simulink library "SLUGS_Library"  (Simulink 7.8)
settings: Solver=ode45  SolverMode=SingleTasking  StartTime=0.0  StopTime=10.0  RelTol=1e-3
values from neighbouring files (symbols this model uses):
  apSampleTime = 0.01    [mcuInit.m]
  derivativesConstant = 5    [mcuInit.m]
  latlong_WP = 1    [mcuInit.m]
  T = 0.01    [mcuInit.m]
  Xpoints = [0 0]    [mcuInit.m]
  Ypoints = [0 0]    [mcuInit.m]
  Zpoints = [0 0]    [mcuInit.m]
undefined symbols (not defined in the file or in its folder): bankCommandLimit, barAdjust, baroCutTemp, baroOffset, baroScale, barTGain1, barTGain2, barTMean1, barTMean2, baseHeight, baseTemp, daLimit, deLimit, DiscIntNeverNeededParam, drLimit, dtLimit, gaind, getGSLocation, getWP, GS_location, Init_onlyOnce, Init_Reset, IPStar, ISA_g, lapseRate, mass, maxAcc, MaxDwnPthStar, maxDynPressure, maxEta, Ndelay, param, pitAdjust, pitchCommandLimit, pitCutTemp, pitotOffset, pitotScale, pitTGain1, pitTGain2, pitTMean1, pitTMean2, polesd, pressureSensorCutoff, rollControlLimit, SampleT, setDiagnosticFloat, setDiagnosticShort, setLogFloat1, setLogFloat2, setNavLong, setNavNav, tanIntercept, Ts, u1, y1, yawDamperLimit, yo, zerosd
libraries: SLUGS_Library x90, simulink x37, dsPICdrivers x33, aerolibconvert2 x4, aerolibutil x1, aerolibobsolete x1
(part 4 of 7)

== system SLUGS_Library/InnerLoop/Longitudinal Channel/Protect NaNs2 ==
  In1 : Inport
  Integer Delay3 : Delay  DelayLength=1  InputProcessing=Inherited  SampleTime=T
  Relational Operator2 : RelationalOperator  Operator===  OutDataTypeStr=uint(8)
  Switch3 : Switch  Criteria=u2 > Threshold  Threshold=0.3  SampleTime=.01
  Out1 : Outport
  wires:
  Relational Operator2/1 -> Switch3/2
  In1/1 -> Switch3/1, Relational Operator2/1, Relational Operator2/2
  Switch3/1 -> Integer Delay3/1, Out1/1
  Integer Delay3/1 -> Switch3/3

== system SLUGS_Library/InnerLoop/Longitudinal Channel/Protect NaNs3 ==
  In1 : Inport
  Integer Delay3 : Delay  DelayLength=1  InputProcessing=Inherited  SampleTime=T
  Relational Operator2 : RelationalOperator  Operator===  OutDataTypeStr=uint(8)
  Switch3 : Switch  Criteria=u2 > Threshold  Threshold=0.3  SampleTime=.01
  Out1 : Outport
  wires:
  Relational Operator2/1 -> Switch3/2
  In1/1 -> Switch3/1, Relational Operator2/1, Relational Operator2/2
  Switch3/1 -> Integer Delay3/1, Out1/1
  Integer Delay3/1 -> Switch3/3

== system SLUGS_Library/InnerLoop/Longitudinal Channel/Protect NaNs4 ==
  In1 : Inport
  Integer Delay3 : Delay  DelayLength=1  InputProcessing=Inherited  SampleTime=T
  Relational Operator2 : RelationalOperator  Operator===  OutDataTypeStr=uint(8)
  Switch3 : Switch  Criteria=u2 > Threshold  Threshold=0.3  SampleTime=.01
  Out1 : Outport
  wires:
  Relational Operator2/1 -> Switch3/2
  In1/1 -> Switch3/1, Relational Operator2/1, Relational Operator2/2
  Switch3/1 -> Integer Delay3/1, Out1/1
  Integer Delay3/1 -> Switch3/3

== system SLUGS_Library/InnerLoop/Longitudinal Channel/Subsystem5 ==
  u : Inport
  C Function Call1 : dsPICdrivers/OTHERS/C Function Call  Tag=dsPIC_dsPIC_CFunctionCall  FctUpdate=Output Function  fctName='myCos'  INPUT_SIZE=1  INPUT1=real32  INPUT2=--  INPUT3=--  OUTPUT_SIZE=1  OUTPUT1=real32  SampleTime=-1  InputType=[ 7 ]  OutputType=[ 7 ]  FctDeclaration=extern real32_T myCos(real32_T u1);  FctCall=%y1 = myCos(%u1);  OrderingInOutPopup=None  FctStart=None  FctStart_Name=Init_onlyOnce  FctStart_Declaration=inline extern void Init_onlyOnce();  FctStart_Call=Init_onlyOnce();  FctInit=None  FctInit_Name=Init_Reset  FctInit_Declaration=inline extern void Init_Reset();  FctInit_Call=Init_Reset();  PinDigitalInput=[]  PinDigitalOutput=[]  AnalogueInput=[]
  cos(u) : Outport
  wires:
  C Function Call1/1 -> cos(u)/1
  u/1 -> C Function Call1/1

== system SLUGS_Library/InnerLoop/Navigation/Compute WP Index ==
  T1 : Inport
  Puav : Inport  Port=2
  Max WP Index : Inport  Port=3
  StartingWP : Inport  Port=4
  "WP1 " : Inport  Port=5
  R : Inport  Port=6
  WP Fly : Inport  Port=7
  Add : Sum  Inputs=2
  Compute Distance : SLUGS_Library/Navigation/Compute Distance
  Compute Modified L1 : Subsystem
  Data Type Conversion : DataTypeConversion  OutDataTypeStr=double  SampleTime=apSampleTime
  Data Type Conversion1 : DataTypeConversion  OutDataTypeStr=double  SampleTime=apSampleTime
  Embedded MATLAB Function : MATLAB Function  TreatAsAtomicUnit=on
  Enabled Subsystem : Subsystem  TreatAsAtomicUnit=on
  Hit  Crossing : HitCross  HitCrossingOffset=0.9  HitCrossingDirection=rising  SampleTime=apSampleTime
  IC : InitialCondition
  IC1 : InitialCondition  Value=0
  Integer Delay : Delay  DelayLength=1  InputProcessing=Inherited
  Integer Delay2 : Delay  DelayLength=1  InitialCondition=0  InputProcessing=Inherited
  Integer Delay3 : Delay  DelayLength=1  InitialCondition=150  InputProcessing=Inherited
  Logical Operator : Logic  Operator=OR  AllPortsSameDT=off  OutDataTypeStr=boolean
  "Puav " : InportShadow  Port=2
  Subsystem : Subsystem
  Switch Distance Less than? : RelationalOperator  OutDataTypeStr=boolean  SampleTime=apSampleTime
  WP1 1 : InportShadow  Port=5
  WP Change : Outport
  WP0 : Outport  Port=2
  WP1 : Outport  Port=3
  UAV IC : Outport  Port=4
  wires:
  [WpEnabl] -> Logical Operator/2
  Logical Operator/1 -> WP Change/1
  [WpEnabl] -> Embedded MATLAB Function/4(wpEnabl)
  IC1/1 -> Subsystem/1(WP Fly)
  Enabled Subsystem/1(Out1) -> UAV IC/1
  "Puav "/1 -> Enabled Subsystem/1(In1)
  Subsystem/1(Just Enab) -> [WpEnabl], Enabled Subsystem/Enable
  WP Fly/1 -> Data Type Conversion1/1
  R/1 -> Compute Modified L1/4(R)
  Integer Delay3/1 -> Switch Distance Less than?/1
  Compute Modified L1/1(P) -> Integer Delay3/1
  IC/1 -> Integer Delay2/1, Add/2
  Add/1 -> Logical Operator/1, Compute Modified L1/Enable
  Integer Delay2/1 -> Add/1
  T1/1 -> Compute Modified L1/2(T1)
  WP1 1/1 -> Compute Modified L1/1(WP1)
  Embedded MATLAB Function/3(wp2) -> Compute Modified L1/3(WP2)
  Data Type Conversion/1 -> Hit  Crossing/1
  Hit  Crossing/1 -> IC/1, Embedded MATLAB Function/3(swIncrement)
  "WP1 "/1 -> Integer Delay/1
  Compute Distance/1 -> Switch Distance Less than?/2
  Max WP Index/1 -> Embedded MATLAB Function/2(wpCount)
  Switch Distance Less than?/1 -> Data Type Conversion/1
  StartingWP/1 -> Embedded MATLAB Function/1(wpStart)
  Embedded MATLAB Function/1(wp0) -> WP0/1
  Embedded MATLAB Function/2(wp1) -> WP1/1
  Puav/1 -> Compute Distance/1
  Integer Delay/1 -> Compute Distance/2  "next WP"
  Data Type Conversion1/1 -> IC1/1

== system SLUGS_Library/InnerLoop/Navigation/Get Wps Compute Frenet ==
  WP Idx 0 : Inport
  WP Idx 1 : Inport  Port=2
  UAV IC : Inport  Port=3
  Enable : EnablePort
  Compute Frenet : SLUGS_Library/Navigation/Compute Frenet
  Switch : Switch  Criteria=u2 > Threshold  Threshold=0.3
  get WP Coord from Index : SLUGS_Library/Navigation/get WP Coord from Index
  "get WP Coord from Index " : SLUGS_Library/Navigation/get WP Coord from Index
  T : Outport
  N : Outport  Port=2
  WP 1 : Outport  Port=3
  wires:
  WP Idx 0/1 -> get WP Coord from Index/1, Switch/2
  Compute Frenet/1 -> T/1
  Compute Frenet/2 -> N/1
  WP Idx 1/1 -> "get WP Coord from Index "/1
  "get WP Coord from Index "/1 -> Compute Frenet/2, WP 1/1
  Switch/1 -> Compute Frenet/1
  get WP Coord from Index/1 -> Switch/1
  UAV IC/1 -> Switch/3

== system SLUGS_Library/Navigation/Compute WP Index/Compute Modified L1 ==
  WP1 : Inport
  T1 : Inport  Port=2
  WP2 : Inport  Port=3
  R : Inport  Port=4
  Enable : EnablePort  ShowOutputPort=on
  Compute T  in Frenet : Subsystem  AncestorBlock=SLUGS_Library/Navigation/Compute Frenet
  Get Circles : Subsystem
  Integer Delay1 : Delay  DelayLength=1  InputProcessing=Inherited
  Integer Delay2 : Delay  DelayLength=1  InputProcessing=Inherited
  To Workspace : ToWorkspace  VariableName=wpChange  SampleTime=-1  SaveFormat=Structure
  WP1_1 : InportShadow  Port=1
  get WP Coord from Index : SLUGS_Library/Navigation/get WP Coord from Index
  P : Outport
  wires:
  get WP Coord from Index/1 -> Integer Delay2/1
  Integer Delay2/1 -> Compute T  in Frenet/2(Pos 2)
  Compute T  in Frenet/1(T) -> Get Circles/2(T2)
  WP1/1 -> Compute T  in Frenet/1(Pos 1)
  WP2/1 -> get WP Coord from Index/1
  T1/1 -> Integer Delay1/1
  Get Circles/1(P) -> P/1
  WP1_1/1 -> Get Circles/3("Wp_to ")
  Integer Delay1/1 -> Get Circles/1(T1)
  Enable/1 -> To Workspace/1
  R/1 -> Get Circles/4(R)

== system SLUGS_Library/Navigation/Compute WP Index/Enabled Subsystem ==
  In1 : Inport
  Enable : EnablePort
  Out1 : Outport
  wires:
  In1/1 -> Out1/1

== system SLUGS_Library/Navigation/Compute WP Index/Subsystem ==
  WP Fly : Inport
  Add1 : Sum  Inputs=2
  Hit  Crossing1 : HitCross  HitCrossingOffset=0.3  HitCrossingDirection=rising  SampleTime=apSampleTime
  Integer Delay1 : Delay  DelayLength=1  InitialCondition=0  InputProcessing=Inherited
  Just Enab : Outport
  wires:
  Integer Delay1/1 -> Add1/1
  Hit  Crossing1/1 -> Add1/2, Integer Delay1/1
  Add1/1 -> Just Enab/1
  WP Fly/1 -> Hit  Crossing1/1

== system SLUGS_Library/Navigation/Geod2LTP/ECEF2LTP (UEN) ==
  ECEF coordinates : Inport
  "Long, Lat" : Inport  Port=2
  Deg2R : Gain  Gain=pi/180  SaturateOnIntegerOverflow=on  OutDataTypeStr=Inherit: Same as input  ParamDataTypeStr=Inherit: Same as input
  Demux3 : Demux  Outputs=2
  From Body to Universal1 : Subsystem
  Product1 : Product  Multiplication=Matrix(*)  SaturateOnIntegerOverflow=on  InputSameDT=on  OutDataTypeStr=Inherit: Same as first input
  Out : Outport
  wires:
  From Body to Universal1/1(DCM) -> Product1/1
  ECEF coordinates/1 -> Product1/2
  Deg2R/1 -> Demux3/1
  Demux3/1 -> From Body to Universal1/1(long)
  Demux3/2 -> From Body to Universal1/2(lat)
  Product1/1 -> Out/1
  "Long, Lat"/1 -> Deg2R/1

== system SLUGS_Library/Navigation/Geod2LTP/Geod2ECEF1 ==
  "height, m" : Inport
  "lat, deg" : Inport  Port=2
  lon,deg : Inport  Port=3
  (Rh+h)cos(phi)*cos(lamb)=Xe : Product  Inputs=3  OutDataTypeStr=single  SaturateOnIntegerOverflow=on  InputSameDT=on
  (Rh+h)cos(phi)*sin(lamb)=Ye : Product  Inputs=3  OutDataTypeStr=single  SaturateOnIntegerOverflow=on  InputSameDT=on
  Deg2R : Gain  Gain=pi/180  OutDataTypeStr=float('single')  SaturateOnIntegerOverflow=on  ParamDataTypeStr=Inherit: Same as input
  Deg2R1 : Gain  Gain=pi/180  OutDataTypeStr=float('single')  SaturateOnIntegerOverflow=on  ParamDataTypeStr=Inherit: Same as input
  Product1 : Product  SaturateOnIntegerOverflow=on  InputSameDT=on  OutDataTypeStr=Inherit: Same as first input
  Re=equatorial radius : Constant  Value=Re  OutDataTypeStr=single
  Rh : Product  Inputs=*/  OutDataTypeStr=single  SaturateOnIntegerOverflow=on  InputSameDT=on
  Rh(1-e^2) : Product  OutDataTypeStr=single  SaturateOnIntegerOverflow=on  InputSameDT=on
  Sum1 : Sum  Inputs=+-|  SaturateOnIntegerOverflow=on  InputSameDT=on  OutDataTypeStr=Inherit: Same as first input
  Sum2 : Sum  SaturateOnIntegerOverflow=on  InputSameDT=on  OutDataTypeStr=Inherit: Same as first input
      settings: AttributesFormatString=Rh+h
  Sum3 : Sum  Inputs=|+-  SaturateOnIntegerOverflow=on  InputSameDT=on  OutDataTypeStr=Inherit: Same as first input
  Sum4 : Sum  OutDataTypeStr=single  SaturateOnIntegerOverflow=on  InputSameDT=on
      settings: AttributesFormatString=(1-e^2)Rh+h
  Ze : Product  OutDataTypeStr=single  SaturateOnIntegerOverflow=on  InputSameDT=on
  const : Constant  OutDataTypeStr=single
  const1 : Constant  OutDataTypeStr=single
  cos(lamb) : Trigonometry  Operator=cos
  cos(phi) : Trigonometry  Operator=cos
  eccentricity^2 : Subsystem
  f : Fcn  Expr=sqrt(u(1))
  sin(lamb) : Trigonometry
  sin(phi) : Trigonometry
  sin(phi)^2 : Product  SaturateOnIntegerOverflow=on  InputSameDT=on  OutDataTypeStr=Inherit: Same as first input
  "Xe, m " : Outport
  "Ye, m " : Outport  Port=2
  "Ze, m " : Outport  Port=3
  wires:
  (Rh+h)cos(phi)*sin(lamb)=Ye/1 -> "Ye, m "/1
  (Rh+h)cos(phi)*cos(lamb)=Xe/1 -> "Xe, m "/1
  Sum2/1 -> (Rh+h)cos(phi)*cos(lamb)=Xe/1, (Rh+h)cos(phi)*sin(lamb)=Ye/1
  Deg2R1/1 -> sin(lamb)/1, cos(lamb)/1
  Deg2R/1 -> sin(phi)/1, cos(phi)/1
  Ze/1 -> "Ze, m "/1
  sin(lamb)/1 -> (Rh+h)cos(phi)*sin(lamb)=Ye/3
  cos(lamb)/1 -> (Rh+h)cos(phi)*cos(lamb)=Xe/3
  cos(phi)/1 -> (Rh+h)cos(phi)*sin(lamb)=Ye/2, (Rh+h)cos(phi)*cos(lamb)=Xe/2
  lon,deg/1 -> Deg2R1/1
  Sum4/1 -> Ze/2
  Rh(1-e^2)/1 -> Sum4/1
  Sum3/1 -> Rh(1-e^2)/1  "1-e^2"
  const1/1 -> Sum3/1
  sin(phi)^2/1 -> Product1/2
  eccentricity^2/1(e^2) -> Sum3/2, Product1/1
  "height, m"/1 -> Sum2/1, Sum4/2
  const/1 -> Sum1/1
  Sum1/1 -> f/1
  Product1/1 -> Sum1/2
  Rh/1 -> Rh(1-e^2)/2, Sum2/2
  Re=equatorial radius/1 -> Rh/1
  f/1 -> Rh/2
  sin(phi)/1 -> Ze/1, sin(phi)^2/2, sin(phi)^2/1
  "lat, deg"/1 -> Deg2R/1

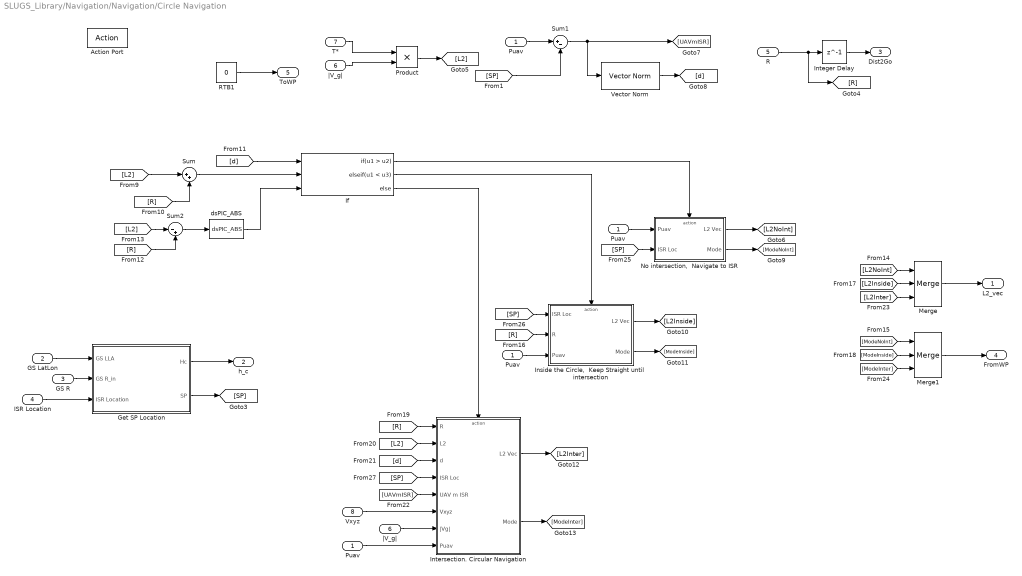
== system SLUGS_Library/Navigation/Navigation/Circle Navigation ==
  Puav : Inport
  GS LatLon : Inport  Port=2
  GS R : Inport  Port=3
  ISR Location : Inport  Port=4
  R : Inport  Port=5
  |V_g| : Inport  Port=6
  T* : Inport  Port=7
  Vxyz : Inport  Port=8
  Action Port : ActionPort
  Get SP Location : Subsystem
  If : If  NumInputs=3  IfExpression=u1 > u2  ElseIfExpressions=u1 < u3
  "Inside the Circle,  Keep Straight until  intersection" : Subsystem  TreatAsAtomicUnit=on
  Integer Delay : Delay  DelayLength=1  InputProcessing=Inherited
  Intersection. Circular Navigation : Subsystem  TreatAsAtomicUnit=on
  Merge : Merge  Inputs=3
  Merge1 : Merge  Inputs=3
  "No intersection,  Navigate to ISR" : Subsystem  TreatAsAtomicUnit=on
  Product : Product  OutDataTypeStr=single  RndMeth=Zero
  "Puav   " : InportShadow  Port=1
  "Puav    " : InportShadow  Port=1
  "Puav     " : InportShadow  Port=1
  RTB1 : Constant  Value=0  OutDataTypeStr=uint8
  Sum : Sum  Inputs=|++
  Sum1 : Sum  Inputs=|+-
  Sum2 : Sum  Inputs=|-+
  Vector Norm : SLUGS_Library/Vector Norm
  dsPIC_ABS : SLUGS_Library/dsPIC_ABS
  "|V_g| " : InportShadow  Port=6
  L2_vec : Outport
  h_c : Outport  Port=2
  Dist2Go : Outport  Port=3
  FromWP : Outport  Port=4  InitialOutput=[1]
  ToWP : Outport  Port=5  InitialOutput=[1]
  wires:
  "Puav     "/1 -> Intersection. Circular Navigation/8(Puav)
  Get SP Location/1(Hc) -> h_c/1
  [ModeInter] -> Merge1/3
  [L2Inter] -> Merge/3
  "|V_g| "/1 -> Intersection. Circular Navigation/7(|Vg|)
  Vxyz/1 -> Intersection. Circular Navigation/6(Vxyz)
  [UAVmISR] -> Intersection. Circular Navigation/5(UAV m ISR)
  [SP] -> Intersection. Circular Navigation/4(ISR Loc)
  [d] -> Intersection. Circular Navigation/3(d)
  [L2] -> Intersection. Circular Navigation/2(L2)
  [R] -> Intersection. Circular Navigation/1(R)
  Intersection. Circular Navigation/2(Mode) -> [ModeInter]
  Intersection. Circular Navigation/1(L2 Vec) -> [L2Inter]
  Puav/1 -> "Inside the Circle,  Keep Straight until  intersection"/3(Puav)
  [ModeInside] -> Merge1/2
  [L2Inside] -> Merge/2
  "Inside the Circle,  Keep Straight until  intersection"/2(Mode) -> [ModeInside]
  "Inside the Circle,  Keep Straight until  intersection"/1(L2 Vec) -> [L2Inside]
  [R] -> "Inside the Circle,  Keep Straight until  intersection"/2(R)
  [SP] -> "Inside the Circle,  Keep Straight until  intersection"/1(ISR Loc)
  [ModeNoInt] -> Merge1/1
  [L2NoInt] -> Merge/1
  "No intersection,  Navigate to ISR"/2(Mode) -> [ModeNoInt]
  "No intersection,  Navigate to ISR"/1(L2 Vec) -> [L2NoInt]
  [SP] -> "No intersection,  Navigate to ISR"/2(ISR Loc)
  "Puav    "/1 -> "No intersection,  Navigate to ISR"/1(Puav)
  If/3 -> Intersection. Circular Navigation/Action
  If/2 -> "Inside the Circle,  Keep Straight until  intersection"/Action
  If/1 -> "No intersection,  Navigate to ISR"/Action
  Merge/1 -> L2_vec/1
  dsPIC_ABS/1 -> If/3
  Sum2/1 -> dsPIC_ABS/1
  [R] -> Sum2/2
  [L2] -> Sum2/1
  Sum/1 -> If/2
  [d] -> If/1
  Vector Norm/1 -> [d]
  Sum1/1 -> [UAVmISR], Vector Norm/1
  [SP] -> Sum1/2
  "Puav   "/1 -> Sum1/1
  [R] -> Sum/2
  [L2] -> Sum/1
  RTB1/1 -> ToWP/1
  T*/1 -> Product/1
  |V_g|/1 -> Product/2
  Product/1 -> [L2]
  Get SP Location/2(SP) -> [SP]
  GS LatLon/1 -> Get SP Location/1(GS LLA)
  GS R/1 -> Get SP Location/2(GS R_in)
  ISR Location/1 -> Get SP Location/3(ISR Location)
  Integer Delay/1 -> Dist2Go/1
  R/1 -> Integer Delay/1, [R]
  Merge1/1 -> FromWP/1

== system SLUGS_Library/Navigation/Navigation/Get 2D Groundspeed ==
  Vxyz : Inport  SampleTime=apSampleTime
  Vector Norm : SLUGS_Library/Vector Norm
  |V_g| : Outport
  wires:
  Vector Norm/1 -> |V_g|/1
  Vxyz/1 -> Vector Norm/1

== system SLUGS_Library/Navigation/Navigation/L2+ ==
  |V_g| : Inport
  L2_vec : Inport  Port=2
  Vxyz : Inport  Port=3
  T*(m) : Inport  Port=4
  Constant10 : Constant  Value=maxEta  OutDataTypeStr=single
  "Get Sin, Cos eta" : Subsystem
  L2+ : Subsystem
  Rad2Deg : Gain  Gain=180/pi
  Relational Operator : RelationalOperator  Operator=<=  OutDataTypeStr=boolean
  Subsystem : Subsystem
  Switch : Switch  Criteria=u2 > Threshold  Threshold=0.3
  dsPIC_ABS : SLUGS_Library/dsPIC_ABS
  dsPIC_atan2 : SLUGS_Library/dsPIC_atan2
  "if sin(eta) < 0 - maxAcc else                 maxAcc " : Subsystem
  "|V_g| " : InportShadow  Port=1
  phi_c : Outport
  eta : Outport  Port=2
  wires:
  Rad2Deg/1 -> eta/1
  Subsystem/1(phi_c) -> phi_c/1
  T*(m)/1 -> L2+/3(T*)
  "|V_g| "/1 -> L2+/2(|V_g|)
  "Get Sin, Cos eta"/1(sin(eta)) -> L2+/1(sin(eta)), dsPIC_atan2/1, "if sin(eta) < 0 - maxAcc else                 maxAcc "/1(sin(eta))
  "Get Sin, Cos eta"/2(cos(eta)) -> dsPIC_atan2/2
  dsPIC_atan2/1 -> Rad2Deg/1, dsPIC_ABS/1  "eta"
  dsPIC_ABS/1 -> Relational Operator/1
  Constant10/1 -> Relational Operator/2
  Relational Operator/1 -> Switch/2
  L2+/1(a_c) -> Switch/1
  "if sin(eta) < 0 - maxAcc else                 maxAcc "/1(+ - maxAcc) -> Switch/3
  Switch/1 -> Subsystem/1(a_c)
  |V_g|/1 -> "Get Sin, Cos eta"/1(|V_g|)
  L2_vec/1 -> "Get Sin, Cos eta"/2(L2_vec)
  Vxyz/1 -> "Get Sin, Cos eta"/3(Vxyz)

== system SLUGS_Library/Navigation/Navigation/Line Segment ==
  Puav : Inport
  MidLvl h_c : Inport  Port=2
  Action Port : ActionPort
  Gain : Gain  Gain=-1
  Gain1 : Gain  Gain=-1
  "Puav " : InportShadow  Port=1
  RTB : Constant  Value=0  OutDataTypeStr=uint8
  RTB1 : Constant  Value=0  OutDataTypeStr=uint8
  Vector Norm : SLUGS_Library/Vector Norm
  L2_vec : Outport
  h_c : Outport  Port=2
  Dist2Go : Outport  Port=3
  FromWP : Outport  Port=4  InitialOutput=[1]
  ToWP : Outport  Port=5  InitialOutput=[2]
  wires:
  Gain/1 -> L2_vec/1
  Puav/1 -> Gain/1
  MidLvl h_c/1 -> h_c/1
  Vector Norm/1 -> Dist2Go/1
  RTB/1 -> FromWP/1
  "Puav "/1 -> Gain1/1
  Gain1/1 -> Vector Norm/1
  RTB1/1 -> ToWP/1

== system SLUGS_Library/Navigation/Navigation/Minimum Turn Radius ==
  U_c : Inport
  Scale Factor : Inport  Port=2
  Constant1 : Constant  Value=maxAcc  OutDataTypeStr=single
  IC : InitialCondition  Value=1.5
  Product1 : Product  RndMeth=Zero
  Product2 : Product  RndMeth=Zero
  Product3 : Product  Inputs=*/  RndMeth=Zero
  "[1.5 10]" : Saturate  UpperLimit=10  LowerLimit=1.5
  R : Outport
  wires:
  U_c/1 -> Product1/2, Product1/1
  Product2/1 -> Product3/1
  Constant1/1 -> Product3/2
  Product1/1 -> Product2/2
  Scale Factor/1 -> IC/1
  Product3/1 -> R/1
  "[1.5 10]"/1 -> Product2/1
  IC/1 -> "[1.5 10]"/1

== system SLUGS_Library/Navigation/Navigation/Normal WP  Navigation ==
  wpEnable : Inport
  GS_LatLon : Inport  Port=2
  GS_R_in : Inport  Port=3
  |V_g| : Inport  Port=4
  T* : Inport  Port=5
  Puav : Inport  Port=6
  TurnLeadTime : Inport  Port=7
  MaxWp : Inport  Port=8
  Action Port : ActionPort
  Add : Sum  Inputs=+-
  Compute WP Switching Trigger : Subsystem
  Constant1 : Constant  OutDataTypeStr=boolean  SampleTime=0.01
  Constant2 : Constant  OutDataTypeStr=boolean  SampleTime=0.01
  Embedded MATLAB Function : MATLAB Function  TreatAsAtomicUnit=on
  "GS_LatLon " : InportShadow  Port=2
  "GS_R_in " : InportShadow  Port=3
  Gain : Gain  Gain=0.4
  Get Frenet : Subsystem
  IC : InitialCondition  Value=0
  Integer Delay : Delay  DelayLength=1  InitialCondition=1  InputProcessing=Inherited
  On WP Enable : Subsystem  TreatAsAtomicUnit=on
  Product : Product  OutDataTypeStr=single  RndMeth=Zero
  "Puav " : InportShadow  Port=6
  Relational Operator : RelationalOperator  Operator=>  OutDataTypeStr=boolean
  Switch : Switch  Criteria=u2 > Threshold  Threshold=0.3  ZeroCross=off
  Switch1 : Switch  Criteria=u2 > Threshold  Threshold=0.3  ZeroCross=off
  To Workspace : ToWorkspace  VariableName=IP  SampleTime=-1  SaveFormat=Array
  To Workspace1 : ToWorkspace  VariableName=L2Vec  SampleTime=-1  SaveFormat=Array
  To Workspace2 : ToWorkspace  VariableName=AimPointVect  SampleTime=-1  SaveFormat=Array
  To Workspace3 : ToWorkspace  VariableName=IPReached  SampleTime=-1  SaveFormat=Array
  Vector Norm : SLUGS_Library/Vector Norm
  Zero out Z2 : MATLAB Function  TreatAsAtomicUnit=on
  computeCurrentWP : MATLAB Function  TreatAsAtomicUnit=on
  "|V_g| " : InportShadow  Port=4
  L2_vec : Outport
  h_c : Outport  Port=2
  Dist2Go : Outport  Port=3
  FromWP : Outport  Port=4  InitialOutput=[1]
  ToWP : Outport  Port=5  InitialOutput=[2]
  wires:
  IC/1 -> Switch/2, To Workspace3/1, [IPReached]
  [L2] -> Compute WP Switching Trigger/6(L2)
  MaxWp/1 -> computeCurrentWP/2(maxWp)
  computeCurrentWP/2(WP1) -> Get Frenet/4(To WP), ToWP/1
  computeCurrentWP/1(WP0) -> Get Frenet/3(From WP), FromWP/1
  Compute WP Switching Trigger/1(Switch) -> Integer Delay/1
  Compute WP Switching Trigger/3(L2Vec) -> To Workspace1/1, Switch/1
  Get Frenet/4(N1) -> Compute WP Switching Trigger/3(N1)
  Get Frenet/5(TurnLeadDistance) -> Compute WP Switching Trigger/4(LeadDistance)
  TurnLeadTime/1 -> Get Frenet/5(TurnLeadTime)
  "|V_g| "/1 -> Get Frenet/6(|V_g|)
  "Puav "/1 -> Add/2
  Puav/1 -> Compute WP Switching Trigger/5(Puav)
  Get Frenet/3(T1) -> Compute WP Switching Trigger/2(T1)
  Get Frenet/2(ToWp) -> Compute WP Switching Trigger/1(ToWp)
  "GS_R_in "/1 -> Get Frenet/2(GS R_in)
  "GS_LatLon "/1 -> Get Frenet/1(GS LLA)
  Embedded MATLAB Function/1(reached) -> IC/1
  Switch/1 -> L2_vec/1
  Relational Operator/1 -> Embedded MATLAB Function/2(didReachIP)
  Vector Norm/1 -> Relational Operator/2, [dist2AP]  "Dist2AimPoint"
  Gain/1 -> Relational Operator/1
  [L2] -> Gain/1
  Add/1 -> To Workspace2/1, Switch/3, Vector Norm/1  "Pa = HP - Pned"
  Zero out Z2/1(P) -> Add/1
  On WP Enable/1(P_i) -> To Workspace/1, Zero out Z2/1(Pin)  "WP0 - L2*IP*T1"
  GS_R_in/1 -> On WP Enable/3(GS R_in)
  GS_LatLon/1 -> On WP Enable/2(GS LLA)
  [L2] -> On WP Enable/1(L2)
  Product/1 -> [L2]
  |V_g|/1 -> Product/2
  T*/1 -> Product/1
  wpEnable/1 -> Embedded MATLAB Function/1(wpEnable)
  [IPReached] -> computeCurrentWP/3(IPReached)
  [IPReached] -> Switch1/2
  Compute WP Switching Trigger/2(Dist2WP1) -> Switch1/1
  Switch1/1 -> Dist2Go/1
  [dist2AP] -> Switch1/3
  Integer Delay/1 -> computeCurrentWP/1(WPSwitch)
  Constant1/1 -> On WP Enable/Enable
  Constant2/1 -> Get Frenet/Enable
  Get Frenet/1(H_c) -> h_c/1

== system SLUGS_Library/Navigation/Navigation/RTB/Follow Mobile Navigation ==
  Mobile Location : Inport
  Follow Mobile? : Inport  Port=2
  MidLvl h_c : Inport  Port=3
  GS LatLon : Inport  Port=4
  GS R : Inport  Port=5
  Puav : Inport  Port=6
  Action Port : ActionPort
  Compute Mobile Location : Subsystem  TreatAsAtomicUnit=on
  Constant : Constant  Value=[0 0 0]  OutDataTypeStr=single
  RTB : Constant  Value=0  OutDataTypeStr=uint8
  RTB1 : Constant  Value=0  OutDataTypeStr=uint8
  Simple Predictor : Subsystem
  Subtract : Sum  Inputs=+-
  Switch : Switch  Threshold=0.3
  To Workspace : ToWorkspace  VariableName=BP  SampleTime=-1  SaveFormat=Array
  Vector Norm : SLUGS_Library/Vector Norm
  Zero out Z1 : MATLAB Function  TreatAsAtomicUnit=on
  L2_vec : Outport
  h_c : Outport  Port=2
  Dist2Go : Outport  Port=3
  FromWP : Outport  Port=4  InitialOutput=[0]
  ToWP : Outport  Port=5  InitialOutput=[0]
  wires:
  MidLvl h_c/1 -> h_c/1
  Zero out Z1/1(P) -> Subtract/1
  Puav/1 -> Subtract/2
  Subtract/1 -> To Workspace/1, Simple Predictor/1(Base Point), Vector Norm/1
  Switch/1 -> Zero out Z1/1(Pin)
  Simple Predictor/1(Predicted Bp) -> L2_vec/1
  Mobile Location/1 -> Compute Mobile Location/1("Lat, Lon")
  GS R/1 -> Compute Mobile Location/3(GS R)
  GS LatLon/1 -> Compute Mobile Location/2(GS LLA)
  Follow Mobile?/1 -> Switch/2, Compute Mobile Location/Enable
  Compute Mobile Location/1(XYZ) -> Switch/1
  Constant/1 -> Switch/3
  Vector Norm/1 -> Dist2Go/1
  RTB/1 -> FromWP/1
  RTB1/1 -> ToWP/1

== system SLUGS_Library/Navigation/Navigation/Recent Enable ==
  WP Fly : Inport
  Grab Upon Enable : Subsystem  TreatAsAtomicUnit=on
  IC1 : InitialCondition  Value=0
  IC2 : InitialCondition  Value=0
  IC3 : InitialCondition  Value=0
  IC4 : InitialCondition  Value=[36.988506 -122.055308]
  Subsystem : Subsystem
  WPEnable : Outport
  "GS, Lat Lon" : Outport  Port=2
  GS R_in : Outport  Port=3
  GS Alt (m) : Outport  Port=4
  wires:
  IC3/1 -> GS Alt (m)/1
  IC4/1 -> "GS, Lat Lon"/1
  Grab Upon Enable/2(GS R_in) -> GS R_in/1
  Grab Upon Enable/1("GS, Lon, Lat") -> IC4/1
  WP Fly/1 -> IC1/1
  Subsystem/1(Just Enab) -> IC2/1, WPEnable/1
  IC1/1 -> Subsystem/1(WP Fly)
  IC2/1 -> Grab Upon Enable/Enable
  Grab Upon Enable/3(GS Altitude (m)) -> IC3/1

== system SLUGS_Library/Navigation/Park, Deyst & How Lat Accel Cmd/Compute Eta ==
  Vxyz : Inport
  L1_vec : Inport  Port=2
  3x3 Cross Product : aerolibutil/3x3 Cross Product
  Divide5 : Product  Inputs=*//
  Norm : SLUGS_Library/Navigation/Norm
  "Norm " : SLUGS_Library/Navigation/Norm
  Selector : Selector  InputPortWidth=3  IndexOptions=Index vector (dialog)  Indices=[3]  OutputSizes=1
  Subsystem6 : SLUGS_Library/Subsystem6
  To Workspace : ToWorkspace  VariableName=L1  SampleTime=-1  SaveFormat=Array
  To Workspace1 : ToWorkspace  VariableName=Vned  SampleTime=-1  SaveFormat=Array
  To Workspace2 : ToWorkspace  VariableName=eta  SampleTime=-1  SaveFormat=Array
  negprotect : MATLAB Function  TreatAsAtomicUnit=on
  negprotect1 : MATLAB Function  TreatAsAtomicUnit=on
  Eta : Outport
  wires:
  Subsystem6/1 -> To Workspace2/1, Eta/1
  Selector/1 -> Subsystem6/1
  Vxyz/1 -> "Norm "/1, To Workspace1/1, 3x3 Cross Product/1
  3x3 Cross Product/1 -> Divide5/1
  Norm/1 -> negprotect/1(val)
  "Norm "/1 -> negprotect1/1(val)
  Divide5/1 -> Selector/1
  L1_vec/1 -> Norm/1, 3x3 Cross Product/2, To Workspace/1
  negprotect1/1(zpVal) -> Divide5/3
  negprotect/1(zpVal) -> Divide5/2

== system SLUGS_Library/Navigation/Park, Deyst & How Lat Accel Cmd/Compute L1 Vector LINE MODE ==
  Pe_lat : Inport
  L1 : Inport  Port=2
  T : Inport  Port=3
  N : Inport  Port=4
  Add : Sum  Inputs=-+
  Add2 : Sum  Inputs=-+
  Divide{,1..3} (4 alike) : Product
  Gain : Gain  Gain=-1
  Subsystem1 : SLUGS_Library/Subsystem1
  Subsystem9 : SLUGS_Library/Subsystem9
  To Workspace3 : ToWorkspace  VariableName=Pey  SampleTime=-1  SaveFormat=Array
  L1_vec : Outport
  wires:
  Subsystem9/1 -> Subsystem1/1
  Add2/1 -> L1_vec/1  "L1_vec"
  Gain/1 -> Divide2/2
  L1/1 -> Divide/1, Divide/2
  Pe_lat/1 -> Gain/1, To Workspace3/1, Divide1/2, Divide1/1
  Divide1/1 -> Add/1
  Divide/1 -> Add/2
  Add/1 -> Subsystem9/1
  Subsystem1/1 -> Divide3/2  "||CD||"
  Divide2/1 -> Add2/1  "N*Pey"
  N/1 -> Divide2/1
  T/1 -> Divide3/1
  Divide3/1 -> Add2/2  "||CD||*T"

== system SLUGS_Library/Navigation/Park, Deyst & How Lat Accel Cmd/Park's Lateral Accel Command ==
  Vxyz : Inport
  L1 : Inport  Port=2
  eta : Inport  Port=3
  Constant : Constant  Value=2
  Norm : SLUGS_Library/Navigation/Norm
  Product : Product  Inputs=***/*  RndMeth=Zero
  Subsystem7 : SLUGS_Library/Subsystem7
  a_s_c : Outport
  wires:
  eta/1 -> Subsystem7/1
  Vxyz/1 -> Norm/1
  Norm/1 -> Product/1, Product/2
  Constant/1 -> Product/3
  L1/1 -> Product/4
  Subsystem7/1 -> Product/5
  Product/1 -> a_s_c/1

== system SLUGS_Library/Navigation/get WP Coord from Index/Get WP from idx SIM ==
  GS LLA : Inport
  GS ECEF : Inport  Port=2
  idx : Inport  Port=3
  Constant : Constant  Value=latlong_WP  OutDataTypeStr=uint8  SampleTime=0.01
  Constant1 : Constant  Value=Ypoints  OutDataTypeStr=double  SampleTime=0.01
  Constant2 : Constant  Value=Xpoints  OutDataTypeStr=double  SampleTime=0.01
  Constant3 : Constant  Value=Zpoints  OutDataTypeStr=double  SampleTime=0.01
  Data Type Conversion : DataTypeConversion  OutDataTypeStr=double
  Data Type Conversion1 : DataTypeConversion  OutDataTypeStr=single
  Demux : Demux  Outputs=3
  Geod2LTP1 : SLUGS_Library/Navigation/Geod2LTP
  Mux : Mux  Inputs=3
  Switch : Switch  Criteria=u2 > Threshold  Threshold=0.3  ZeroCross=off
  Zero out Z1 : MATLAB Function  TreatAsAtomicUnit=on
  Zero out Z2 : MATLAB Function  TreatAsAtomicUnit=on
  Zero out Z3 : MATLAB Function  TreatAsAtomicUnit=on
  Out1 : Outport
  wires:
  Data Type Conversion/1 -> Zero out Z2/1(idx), Zero out Z1/1(idx), Zero out Z3/1(idx)
  Zero out Z2/1(y) -> Mux/1
  Zero out Z1/1(y) -> Mux/2
  Zero out Z3/1(y) -> Mux/3
  Mux/1 -> Data Type Conversion1/1
  Constant/1 -> Switch/2
  Demux/1 -> Geod2LTP1/3
  Demux/2 -> Geod2LTP1/4
  Demux/3 -> Geod2LTP1/5
  Geod2LTP1/1 -> Switch/1
  Data Type Conversion1/1 -> Switch/3, Demux/1
  GS LLA/1 -> Geod2LTP1/1
  GS ECEF/1 -> Geod2LTP1/2
  idx/1 -> Data Type Conversion/1
  Switch/1 -> Out1/1
  Constant1/1 -> Zero out Z1/2(vect)
  Constant3/1 -> Zero out Z3/2(vect)
  Constant2/1 -> Zero out Z2/2(vect)

== system SLUGS_Library/Sensor Blocks/Baro Alt/Baro Altimeter ==
  Static (Pa) : Inport
  Compute Barometric Height : Subsystem  mask{baseTemp=baseTemp, LapseRate=lapseRate}
      mask prompts: baseTemp "Base Station Temperature (K)"; LapseRate "Lapse Rate (C/ft)"
      mask help:
      | Produces Altitude in meters from Barometric Pressure in Pascals. Altitude is valid from MSL to 6000 ft.
      |
      | The method implemented here was developed by Ren Curry
  Enabled Subsystem : Subsystem  TreatAsAtomicUnit=on
  Enables/Disables the Computation of  initial Baro Bias : MATLAB Function  TreatAsAtomicUnit=on
  GS Height : Subsystem
  Initial Baro Bias : Subsystem  TreatAsAtomicUnit=on
  Logical Operator : Logic  Operator=NOT  AllPortsSameDT=off  OutDataTypeStr=boolean
  Sum1 : Sum  Inputs=++|  OutDataTypeStr=single
  Zero Out Height : Subsystem  TreatAsAtomicUnit=on
  Altitude : Outport
  wires:
  Compute Barometric Height/1("Altitude, m") -> Zero Out Height/2(Computed Height), Sum1/2
  Static (Pa)/1 -> Initial Baro Bias/1(Baro (Pa)), Compute Barometric Height/3(Baro (Pa))
  Enables/Disables the Computation of  initial Baro Bias/1(tOut) -> Initial Baro Bias/Enable, Zero Out Height/Enable, Logical Operator/1
  GS Height/1(GS Height) -> Compute Barometric Height/1(Base Height (m)), Zero Out Height/1(Base Height)
  Initial Baro Bias/1(Baro (Gnd)) -> Compute Barometric Height/2(Base Pressure (Pa))
  Zero Out Height/1(Height Offset) -> Sum1/1
  Logical Operator/1 -> Enabled Subsystem/Enable
  Sum1/1 -> Enabled Subsystem/1(In1)
  Enabled Subsystem/1(Out1) -> Altitude/1

== system SLUGS_Library/Sensor Blocks/Baro Alt/Barometer Unit Conversion ==
  Raw : Inport
  Bias : Constant  Value=bias  OutDataTypeStr=single
  Divide : Product  OutDataTypeStr=single
  Gains : Constant  Value=gains  OutDataTypeStr=single
  Sum : Sum  Inputs=|++  OutDataTypeStr=single
  Comp : Outport
  wires:
  Bias/1 -> Sum/2
  Raw/1 -> Divide/2
  Gains/1 -> Divide/1
  Divide/1 -> Sum/1
  Sum/1 -> Comp/1

== system SLUGS_Library/Sensor Blocks/Baro Alt/Temp Compensate Baro ==
  Temp : Inport
  Baro : Inport  Port=2
  Compare To Constant : simulink/Logic and Bit Operations/Compare To Constant  relop=<  const=baroCutTemp  OutDataTypeStr=uint8  ZeroCross=off
  Hi Temp Compensation : Subsystem  mask{alpha=barTGain2, tempMean=barTMean2}
      mask prompts: alpha "Tempearature Coeficient (K_t)"; tempMean "Calibration Temperature Mean (T_avg)"
      mask help:
      | This block implements a temperature compensation. It implmements the following equation:
      |
      | M_tc = M_raw - K_t(T - T_avg)
  Lo Temp Compensation : Subsystem  mask{alpha=barTGain1, tempMean=barTMean1}
      mask prompts: alpha "Tempearature Coeficient (K_t)"; tempMean "Calibration Temperature Mean (T_avg)"
      mask help:
      | This block implements a temperature compensation. It implmements the following equation:
      |
      | M_tc = M_raw - K_t(T - T_avg)
  Logical Operator : Logic  Operator=NOT  AllPortsSameDT=off  OutDataTypeStr=boolean
  Merge : Merge
  Baro_c : Outport
  wires:
  Compare To Constant/1 -> Logical Operator/1, Lo Temp Compensation/Enable
  Temp/1 -> Compare To Constant/1, Hi Temp Compensation/2(Temp Raw), Lo Temp Compensation/2(Temp Raw)
  Baro/1 -> Hi Temp Compensation/1(Raw), Lo Temp Compensation/1(Raw)
  Lo Temp Compensation/1(Comp) -> Merge/2
  Merge/1 -> Baro_c/1
  Logical Operator/1 -> Hi Temp Compensation/Enable
  Hi Temp Compensation/1(Comp) -> Merge/1

== system SLUGS_Library/Sensor Blocks/Baro Alt/Tustin Lowpass, Auto Initial Condition ==
  In1 : Inport
  Constant : Constant  Value=T
  Constant1 : Constant  Value=f
  Embedded MATLAB Function : MATLAB Function  TreatAsAtomicUnit=on
  Out1 : Outport
  wires:
  In1/1 -> Embedded MATLAB Function/1(u)
  Embedded MATLAB Function/1(y) -> Out1/1
  Constant1/1 -> Embedded MATLAB Function/3(f)
  Constant/1 -> Embedded MATLAB Function/2(T)

== system SLUGS_Library/Sensor Blocks/Pitot Control End/ 0.3 sec tau for high speeds ==
  In1 : Inport
  Constant : Constant  Value=T
  Constant1 : Constant  Value=f
  Embedded MATLAB Function : MATLAB Function  TreatAsAtomicUnit=on
  Out1 : Outport
  wires:
  In1/1 -> Embedded MATLAB Function/1(u)
  Embedded MATLAB Function/1(y) -> Out1/1
  Constant1/1 -> Embedded MATLAB Function/3(f)
  Constant/1 -> Embedded MATLAB Function/2(T)

== system SLUGS_Library/Sensor Blocks/Pitot Control End/Air Density from Height ==
  h(m) : Inport
  Add : Sum  Inputs=+-
  Constant : Constant  OutDataTypeStr=single
  Constant 2 from Model : Constant  Value=4.255876  OutDataTypeStr=single
  Constant from Model : Constant  Value=145442  OutDataTypeStr=single
  Divide : Product  Inputs=*/
  Divide1 : Product
  Length Conversion : aerolibconvert2/Length Conversion  IU=m  OU=ft
  Rho_0 (Kg/m^3) : Constant  Value=1.225  OutDataTypeStr=single
  "[0 1000]" : Saturate  UpperLimit=1000  LowerLimit=0
  dsPIC Power : SLUGS_Library/dsPIC Power
  rho (Kg/m^3) : Outport
  wires:
  "[0 1000]"/1 -> Length Conversion/1
  dsPIC Power/1 -> Divide1/1
  Constant 2 from Model/1 -> dsPIC Power/2
  Add/1 -> dsPIC Power/1
  Length Conversion/1 -> Divide/1
  Divide1/1 -> rho (Kg/m^3)/1
  Rho_0 (Kg/m^3)/1 -> Divide1/2
  Constant from Model/1 -> Divide/2
  h(m)/1 -> "[0 1000]"/1
  Divide/1 -> Add/2
  Constant/1 -> Add/1

== system SLUGS_Library/Sensor Blocks/Pitot Control End/Compute Airspeed ==
  Dyn P : Inport
  rho : Inport  Port=2
  Divide2 : Product  Inputs=**/
  "[ 0.01 50000]" : Saturate  UpperLimit=50000  LowerLimit=0.01
  a : Constant  Value=2  OutDataTypeStr=single
  dsPIC_SQRT : SLUGS_Library/dsPIC_SQRT
  Airspeed m(s) : Outport
  wires:
  Divide2/1 -> dsPIC_SQRT/1
  dsPIC_SQRT/1 -> Airspeed m(s)/1
  a/1 -> Divide2/1
  Dyn P/1 -> Divide2/2
  rho/1 -> "[ 0.01 50000]"/1
  "[ 0.01 50000]"/1 -> Divide2/3

== system SLUGS_Library/Sensor Blocks/Pitot Control End/Protect NaN ==
  In1 : Inport
  Integer Delay3 : Delay  DelayLength=1  InputProcessing=Inherited  SampleTime=T
  Relational Operator2 : RelationalOperator  Operator===  OutDataTypeStr=uint(8)
  Switch3 : Switch  Criteria=u2 > Threshold  Threshold=0.3  SampleTime=.01
  Out1 : Outport
  wires:
  Relational Operator2/1 -> Switch3/2
  In1/1 -> Switch3/1, Relational Operator2/1, Relational Operator2/2
  Switch3/1 -> Integer Delay3/1, Out1/1
  Integer Delay3/1 -> Switch3/3

== system SLUGS_Library/Sensor Blocks/Pitot Sensor End/Pitot Unit Conversion ==
  Raw : Inport
  Bias : Constant  Value=bias  OutDataTypeStr=single
  Divide : Product  OutDataTypeStr=single
  Gains : Constant  Value=gains  OutDataTypeStr=single
  Sum : Sum  Inputs=|++  OutDataTypeStr=single
  Comp : Outport
  wires:
  Bias/1 -> Sum/2
  Raw/1 -> Divide/2
  Gains/1 -> Divide/1
  Divide/1 -> Sum/1
  Sum/1 -> Comp/1

== system SLUGS_Library/Sensor Blocks/Pitot Sensor End/Temp Compensate Accel X1 ==
  Temp : Inport
  Dynamic : Inport  Port=2
  Compare To Constant : simulink/Logic and Bit Operations/Compare To Constant  relop=<  const=pitCutTemp  OutDataTypeStr=uint8  ZeroCross=off
  Display : Display
  Display2 : Display
  Hi Temp Compensation2 : Subsystem  mask{alpha=pitTGain2, tempMean=pitTMean2}
      mask prompts: alpha "Tempearature Coeficient (K_t)"; tempMean "Calibration Temperature Mean (T_avg)"
      mask help:
      | This block implements a temperature compensation. It implmements the following equation:
      |
      | M_tc = M_raw - K_t(T - T_avg)
  Lo Temp Compensation : Subsystem  mask{alpha=pitTGain1, tempMean=pitTMean1}
      mask prompts: alpha "Tempearature Coeficient (K_t)"; tempMean "Calibration Temperature Mean (T_avg)"
      mask help:
      | This block implements a temperature compensation. It implmements the following equation:
      |
      | M_tc = M_raw - K_t(T - T_avg)
  Logical Operator : Logic  Operator=NOT  AllPortsSameDT=off  OutDataTypeStr=boolean
  Merge : Merge
  Baro_c : Outport
  wires:
  Hi Temp Compensation2/1(Comp) -> Merge/1
  Logical Operator/1 -> Hi Temp Compensation2/Enable, Display2/1
  Merge/1 -> Baro_c/1, Display/1
  Dynamic/1 -> Lo Temp Compensation/1(Raw), Hi Temp Compensation2/1(Raw)
  Temp/1 -> Compare To Constant/1, Lo Temp Compensation/2(Temp Raw), Hi Temp Compensation2/2(Temp Raw)
  Compare To Constant/1 -> Lo Temp Compensation/Enable, Logical Operator/1
  Lo Temp Compensation/1(Comp) -> Merge/2

== system SLUGS_Library/Sensor Blocks/Pitot Sensor End/Tustin Lowpass, Auto Initial Condition3 ==
  In1 : Inport
  Constant : Constant  Value=T
  Constant1 : Constant  Value=f
  Embedded MATLAB Function : MATLAB Function  TreatAsAtomicUnit=on
  Out1 : Outport
  wires:
  Constant/1 -> Embedded MATLAB Function/2(T)
  Constant1/1 -> Embedded MATLAB Function/3(f)
  Embedded MATLAB Function/1(y) -> Out1/1
  In1/1 -> Embedded MATLAB Function/1(u)

== system SLUGS_Library/Singnal Routing & Conditioning/3D Filter/Filter1 ==
  In1 : Inport
  Discrete Zero-Pole : DiscreteZeroPole  Zeros=zerosd  Poles=polesd  Gain=gaind  SampleTime=SampleTime
  Out1 : Outport
  wires:
  In1/1 -> Discrete Zero-Pole/1
  Discrete Zero-Pole/1 -> Out1/1

== system SLUGS_Library/Singnal Routing & Conditioning/3D Filter/Filter2 ==
  In1 : Inport
  Discrete Zero-Pole : DiscreteZeroPole  Zeros=zerosd  Poles=polesd  Gain=gaind  SampleTime=SampleTime
  Out1 : Outport
  wires:
  Discrete Zero-Pole/1 -> Out1/1
  In1/1 -> Discrete Zero-Pole/1

== system SLUGS_Library/Singnal Routing & Conditioning/3D Filter/Filter3 ==
  In1 : Inport
  Discrete Zero-Pole : DiscreteZeroPole  Zeros=zerosd  Poles=polesd  Gain=gaind  SampleTime=SampleTime
  Out1 : Outport
  wires:
  In1/1 -> Discrete Zero-Pole/1
  Discrete Zero-Pole/1 -> Out1/1

== system SLUGS_Library/Singnal Routing & Conditioning/3D LowPass w/Initial Condition/Discrete Low Pass ==
  U : Inport
  Gain : Gain  Gain=(2-a*Ts)  SampleTime=Ts
  Gain1 : Gain  Gain=1/(2+a*Ts)  SampleTime=Ts
  Gain2 : Gain  Gain=a*Ts  SampleTime=Ts
  Sum : Sum  Inputs=++|
  Sum1 : Sum  Inputs=|++
  Unit Delay : UnitDelay  X0=Yo  SampleTime=Ts
  Unit Delay1 : UnitDelay  X0=Yo  SampleTime=Ts
  Y : Outport
  wires:
  Gain/1 -> Sum1/2
  Sum1/1 -> Gain1/1
  Gain2/1 -> Sum1/1
  Gain1/1 -> Y/1, Unit Delay/1  "Y_k"
  Sum/1 -> Gain2/1
  Unit Delay1/1 -> Sum/2  "U_k-1"
  U/1 -> Sum/1, Unit Delay1/1  "U_k"
  Unit Delay/1 -> Gain/1  "Y_k-1"

== system SLUGS_Library/Singnal Routing & Conditioning/3D LowPass w/Initial Condition/Discrete Low Pass1 ==
  U : Inport
  Gain : Gain  Gain=(2-a*Ts)  SampleTime=Ts
  Gain1 : Gain  Gain=1/(2+a*Ts)  SampleTime=Ts
  Gain2 : Gain  Gain=a*Ts  SampleTime=Ts
  Sum : Sum  Inputs=++|
  Sum1 : Sum  Inputs=|++
  Unit Delay : UnitDelay  X0=Yo  SampleTime=Ts
  Unit Delay1 : UnitDelay  X0=Yo  SampleTime=Ts
  Y : Outport
  wires:
  Gain/1 -> Sum1/2
  Sum1/1 -> Gain1/1
  Gain2/1 -> Sum1/1
  Gain1/1 -> Y/1, Unit Delay/1  "Y_k"
  Sum/1 -> Gain2/1
  Unit Delay1/1 -> Sum/2  "U_k-1"
  U/1 -> Sum/1, Unit Delay1/1  "U_k"
  Unit Delay/1 -> Gain/1  "Y_k-1"

== system SLUGS_Library/Singnal Routing & Conditioning/3D LowPass w/Initial Condition/Discrete Low Pass2 ==
  U : Inport
  Gain : Gain  Gain=(2-a*Ts)  SampleTime=Ts
  Gain1 : Gain  Gain=1/(2+a*Ts)  SampleTime=Ts
  Gain2 : Gain  Gain=a*Ts  SampleTime=Ts
  Sum : Sum  Inputs=++|
  Sum1 : Sum  Inputs=|++
  Unit Delay : UnitDelay  X0=Yo  SampleTime=Ts
  Unit Delay1 : UnitDelay  X0=Yo  SampleTime=Ts
  Y : Outport
  wires:
  Gain/1 -> Sum1/2
  Sum1/1 -> Gain1/1
  Gain2/1 -> Sum1/1
  Gain1/1 -> Y/1, Unit Delay/1  "Y_k"
  Sum/1 -> Gain2/1
  Unit Delay1/1 -> Sum/2  "U_k-1"
  U/1 -> Sum/1, Unit Delay1/1  "U_k"
  Unit Delay/1 -> Gain/1  "Y_k-1"

== system SLUGS_Library/Singnal Routing & Conditioning/Ellipse Correction/Subsystem1 ==
  u : Inport
  C Function Call : dsPICdrivers/OTHERS/C Function Call  Tag=dsPIC_dsPIC_CFunctionCall  FctUpdate=Output Function  fctName='mySin'  INPUT_SIZE=1  INPUT1=real32  INPUT2=--  INPUT3=--  OUTPUT_SIZE=1  OUTPUT1=real32  SampleTime=-1  InputType=[ 7 ]  OutputType=[ 7 ]  FctDeclaration=extern real32_T mySin(real32_T u1);  FctCall=%y1 = mySin(%u1);  OrderingInOutPopup=None  FctStart=None  FctStart_Name=Init_onlyOnce  FctStart_Declaration=inline extern void Init_onlyOnce();  FctStart_Call=Init_onlyOnce();  FctInit=None  FctInit_Name=Init_Reset  FctInit_Declaration=inline extern void Init_Reset();  FctInit_Call=Init_Reset();  PinDigitalInput=[]  PinDigitalOutput=[]  AnalogueInput=[]
  C Function Call1 : dsPICdrivers/OTHERS/C Function Call  Tag=dsPIC_dsPIC_CFunctionCall  FctUpdate=Output Function  fctName='myCos'  INPUT_SIZE=1  INPUT1=real32  INPUT2=--  INPUT3=--  OUTPUT_SIZE=1  OUTPUT1=real32  SampleTime=-1  InputType=[ 7 ]  OutputType=[ 7 ]  FctDeclaration=extern real32_T myCos(real32_T u1);  FctCall=%y1 = myCos(%u1);  OrderingInOutPopup=None  FctStart=None  FctStart_Name=Init_onlyOnce  FctStart_Declaration=inline extern void Init_onlyOnce();  FctStart_Call=Init_onlyOnce();  FctInit=None  FctInit_Name=Init_Reset  FctInit_Declaration=inline extern void Init_Reset();  FctInit_Call=Init_Reset();  PinDigitalInput=[]  PinDigitalOutput=[]  AnalogueInput=[]
  sin(u) : Outport
  cos(u) : Outport  Port=2
  wires:
  C Function Call1/1 -> cos(u)/1
  C Function Call/1 -> sin(u)/1
  u/1 -> C Function Call1/1, C Function Call/1

== system SLUGS_Library/Singnal Routing & Conditioning/Ellipse Correction/Subsystem5 ==
  u : Inport
  C Function Call : dsPICdrivers/OTHERS/C Function Call  Tag=dsPIC_dsPIC_CFunctionCall  FctUpdate=Output Function  fctName='mySin'  INPUT_SIZE=1  INPUT1=real32  INPUT2=--  INPUT3=--  OUTPUT_SIZE=1  OUTPUT1=real32  SampleTime=-1  InputType=[ 7 ]  OutputType=[ 7 ]  FctDeclaration=extern real32_T mySin(real32_T u1);  FctCall=%y1 = mySin(%u1);  OrderingInOutPopup=None  FctStart=None  FctStart_Name=Init_onlyOnce  FctStart_Declaration=inline extern void Init_onlyOnce();  FctStart_Call=Init_onlyOnce();  FctInit=None  FctInit_Name=Init_Reset  FctInit_Declaration=inline extern void Init_Reset();  FctInit_Call=Init_Reset();  PinDigitalInput=[]  PinDigitalOutput=[]  AnalogueInput=[]
  C Function Call1 : dsPICdrivers/OTHERS/C Function Call  Tag=dsPIC_dsPIC_CFunctionCall  FctUpdate=Output Function  fctName='myCos'  INPUT_SIZE=1  INPUT1=real32  INPUT2=--  INPUT3=--  OUTPUT_SIZE=1  OUTPUT1=real32  SampleTime=-1  InputType=[ 7 ]  OutputType=[ 7 ]  FctDeclaration=extern real32_T myCos(real32_T u1);  FctCall=%y1 = myCos(%u1);  OrderingInOutPopup=None  FctStart=None  FctStart_Name=Init_onlyOnce  FctStart_Declaration=inline extern void Init_onlyOnce();  FctStart_Call=Init_onlyOnce();  FctInit=None  FctInit_Name=Init_Reset  FctInit_Declaration=inline extern void Init_Reset();  FctInit_Call=Init_Reset();  PinDigitalInput=[]  PinDigitalOutput=[]  AnalogueInput=[]
  sin(u) : Outport
  cos(u) : Outport  Port=2
  wires:
  u/1 -> C Function Call/1, C Function Call1/1
  C Function Call/1 -> sin(u)/1
  C Function Call1/1 -> cos(u)/1

== system SLUGS_Library/Singnal Routing & Conditioning/Ellipse Correction/Subsystem8 ==
  x : Inport
  C Function Call : dsPICdrivers/OTHERS/C Function Call  Tag=dsPIC_dsPIC_CFunctionCall  FctUpdate=Output Function  fctName='myTan'  INPUT_SIZE=1  INPUT1=real32  INPUT2=--  INPUT3=--  OUTPUT_SIZE=1  OUTPUT1=real32  SampleTime=-1  InputType=[ 7 ]  OutputType=[ 7 ]  FctDeclaration=extern real32_T myTan(real32_T u1);  FctCall=%y1 = myTan(%u1);  OrderingInOutPopup=None  FctStart=None  FctStart_Name=Init_onlyOnce  FctStart_Declaration=inline extern void Init_onlyOnce();  FctStart_Call=Init_onlyOnce();  FctInit=None  FctInit_Name=Init_Reset  FctInit_Declaration=inline extern void Init_Reset();  FctInit_Call=Init_Reset();  PinDigitalInput=[]  PinDigitalOutput=[]  AnalogueInput=[]
  tan(x) : Outport
  wires:
  C Function Call/1 -> tan(x)/1
  x/1 -> C Function Call/1

== system SLUGS_Library/Control Blocks/Control Blocks Examples/PD Controller  Internal Derivative/Low_passed Time Derivative ==
  f(t) : Inport
  Add : Sum  Inputs=+-
  Constant : Constant  Value=NDelay*TSample  OutDataTypeStr=single
  Divide : Product  Inputs=*/
  Integer Delay : Delay  DelayLength=NDelay  InputProcessing=Inherited  SampleTime=TSample
  f_dot(t) : Outport
  wires:
  Divide/1 -> f_dot(t)/1
  Constant/1 -> Divide/2
  Integer Delay/1 -> Add/2
  f(t)/1 -> Integer Delay/1, Add/1
  Add/1 -> Divide/1

== system SLUGS_Library/Control Blocks/Control Blocks Examples/PI Controller w/Anti-Windup/Trapezoidal Integrator ==
  x : Inport
  Reset : Inport  Port=2
  Constant : Constant  Value=1/3  OutDataTypeStr=single
  Constant1 : Constant  Value=4/3  OutDataTypeStr=single
  Constant2 : Constant  Value=T/2  OutDataTypeStr=single
  Constant3 : Constant  Value=1/3  OutDataTypeStr=single
  Constant5 : Constant  Value=0  OutDataTypeStr=single
  Integer Delay : Delay  DelayLength=1  InputProcessing=Inherited  SampleTime=T
  Integer Delay1 : Delay  InputProcessing=Inherited  SampleTime=T
  Integer Delay2 : Delay  DelayLength=1  InputProcessing=Inherited  SampleTime=T
  Product{,1..3} (4 alike) : Product  OutDataTypeStr=single  RndMeth=Zero
  Protect NaNs : Subsystem
  "Protect NaNs " : Subsystem
  Subtract : Sum  Inputs=3  OutDataTypeStr=single
  Subtract1 : Sum  Inputs=2  OutDataTypeStr=single
  Switch1 : Switch  Criteria=u2 > Threshold  Threshold=0.3  SampleTime=.01
  Int(x) : Outport
  wires:
  Constant/1 -> Product/2
  Constant1/1 -> Product1/2
  Integer Delay/1 -> Product1/1
  Integer Delay1/1 -> Product2/1
  Constant3/1 -> Product2/2
  x/1 -> "Protect NaNs "/1(In1)
  Product/1 -> Subtract/1
  Product1/1 -> Subtract/2
  Product2/1 -> Subtract/3
  Constant2/1 -> Product3/1
  Subtract/1 -> Product3/2
  Subtract1/1 -> Switch1/3
  Integer Delay2/1 -> Subtract1/1
  Product3/1 -> Subtract1/2
  Constant5/1 -> Switch1/1
  Reset/1 -> Switch1/2
  Switch1/1 -> Protect NaNs/1(In1)
  Protect NaNs/1(Out1) -> Int(x)/1, Integer Delay2/1
  "Protect NaNs "/1(Out1) -> Product/1, Integer Delay/1, Integer Delay1/1

== system SLUGS_Library/Control Blocks/Control Blocks Examples/PID Controller/Low_passed Time Derivative ==
  f(t) : Inport
  Add : Sum  Inputs=+-
  Constant : Constant  Value=NDelay*TSample  OutDataTypeStr=single
  Divide : Product  Inputs=*/  OutDataTypeStr=single
  Integer Delay : Delay  DelayLength=NDelay  InputProcessing=Inherited  SampleTime=TSample
  f_dot(t) : Outport
  wires:
  Add/1 -> Divide/1
  f(t)/1 -> Add/1, Integer Delay/1
  Integer Delay/1 -> Add/2
  Constant/1 -> Divide/2
  Divide/1 -> f_dot(t)/1

== system SLUGS_Library/Control Blocks/Control Blocks Examples/PID Controller w/Anti-Windup/Trapezoidal Integrator ==
  x : Inport
  Reset : Inport  Port=2
  Constant : Constant  Value=1/3  OutDataTypeStr=single
  Constant1 : Constant  Value=4/3  OutDataTypeStr=single
  Constant2 : Constant  Value=T/2  OutDataTypeStr=single
  Constant3 : Constant  Value=1/3  OutDataTypeStr=single
  Constant5 : Constant  Value=0  OutDataTypeStr=single
  Integer Delay : Delay  DelayLength=1  InputProcessing=Inherited  SampleTime=T
  Integer Delay1 : Delay  InputProcessing=Inherited  SampleTime=T
  Integer Delay2 : Delay  DelayLength=1  InputProcessing=Inherited  SampleTime=T
  Product{,1..3} (4 alike) : Product  OutDataTypeStr=single  RndMeth=Zero
  "Protect NaNs " : Subsystem
  Protect NaNs1 : Subsystem
  Subtract : Sum  Inputs=3  OutDataTypeStr=single
  Subtract1 : Sum  Inputs=2  OutDataTypeStr=single
  Switch1 : Switch  Criteria=u2 > Threshold  Threshold=0.3  SampleTime=.01
  Int(x) : Outport
  wires:
  Switch1/1 -> Protect NaNs1/1(In1)
  Reset/1 -> Switch1/2
  Constant5/1 -> Switch1/1
  Product3/1 -> Subtract1/2
  Integer Delay2/1 -> Subtract1/1
  Subtract1/1 -> Switch1/3
  Subtract/1 -> Product3/2
  Constant2/1 -> Product3/1
  Product2/1 -> Subtract/3
  Product1/1 -> Subtract/2
  Product/1 -> Subtract/1
  x/1 -> "Protect NaNs "/1(In1)
  Constant3/1 -> Product2/2
  Integer Delay1/1 -> Product2/1
  Integer Delay/1 -> Product1/1
  Constant1/1 -> Product1/2
  Constant/1 -> Product/2
  Protect NaNs1/1(Out1) -> Integer Delay2/1, Int(x)/1
  "Protect NaNs "/1(Out1) -> Integer Delay1/1, Integer Delay/1, Product/1
